simulink library "annVNC"  (R2022b)
settings: Solver=VariableStepAuto  StartTime=0.0  StopTime=10.0  RelTol=1e-3
undefined symbols (not defined in the file or in its folder): L
libraries: AnnVncBtc x1
settings Model: Creator=darshana.mistry  LastModifiedBy=kl13806
settings SolverCC: AlgebraicLoopSolver=TrustRegion
settings DebuggingCC: UnconnectedInputMsg=warning  UnconnectedOutputMsg=warning  UnconnectedLineMsg=warning  SFMachineParentedDataDiag=warning  ArithmeticOperatorsInVariantConditions=warning
settings ModelReferenceCC: EnableRefExpFcnMdlSchedulingChecks=on
settings SFSimCC: CustomCodeUndefinedFunction=UseInterfaceOnly
settings RTWCC: DLArmComputeVersion=19.05

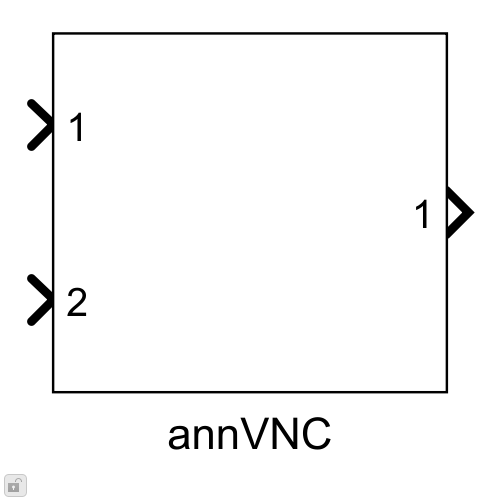
[thumbnail: Simulink's stored preview of the top-level diagram]
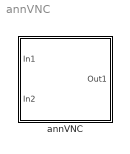
== system annVNC ==
  annVNC : Subsystem  mask{L=L, f_lpf=20, fs_lpf=48000, num=0, den=0, zinit=0}
      mask prompts: L "FrameSize"; f_lpf "Low pass frequency for gain smoothing (Hz)"; fs_lpf "Sampling frequency of LPF"; num "Filter Numerator"; den "Filter Denominator"; zinit "Initial condition"
      mask init:
      | blkh = gcbh;
      | % Copy discrete mask parameters into a classdef object
      | InnerLinkConfig = AnnVncConfig;
      | InnerLinkConfig.FrameSize = L;
      | InnerLinkConfig.LowPassSmoothingHz = f_lpf;
      | InnerLinkConfig.LowPassSamplingHz = fs_lpf;

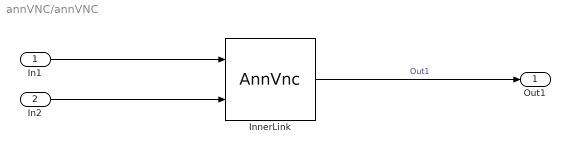
== system annVNC/annVNC ==
  In1 : Inport
  In2 : Inport  Port=2
  InnerLink : AnnVncBtc/AnnVnc  Config=InnerLinkConfig  FeatureName=VNC
      settings: SourceProductName=Bose Blocklib
  Out1 : Outport
  wires:
  InnerLink/1 -> Out1/1  "Out1"
  In1/1 -> InnerLink/1
  In2/1 -> InnerLink/2
